simulink model "bp_attitude_control"  (R2024b)
settings: Solver=FixedStepAuto  StartTime=0.0  StopTime=1000  FixedStep=1  RelTol=1e-3
values from neighbouring files (symbols this model uses):
  H0 = [30; 30; 30]    [initialcondition.m]
  I = [1759 0 0; 0 2758 0; 0 0 2171]    [initialcondition.m]
  qZYX = eul2quat(Euler0)    [initialcondition.m]
  w0 = [0; 0; 0]    [initialcondition.m]
settings Model: Creator=ThinkBook  LastModifiedBy=Lzy18
settings DebuggingCC: UnconnectedInputMsg=warning  UnconnectedOutputMsg=warning  UnconnectedLineMsg=warning
settings ModelReferenceCC: EnableRefExpFcnMdlSchedulingChecks=on
settings RTWCC: GPUComputeCapability=3.5  DLArmComputeVersion=19.05

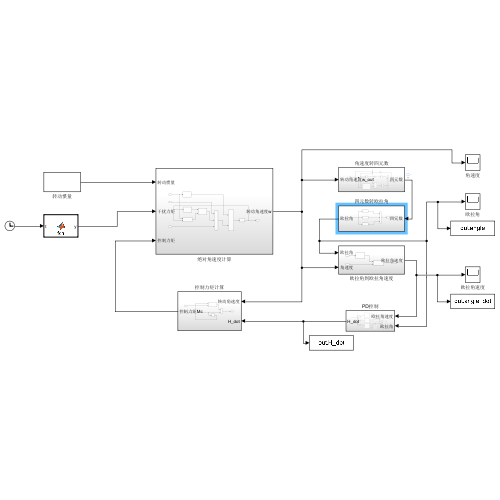
[thumbnail: Simulink's stored preview of the top-level diagram]
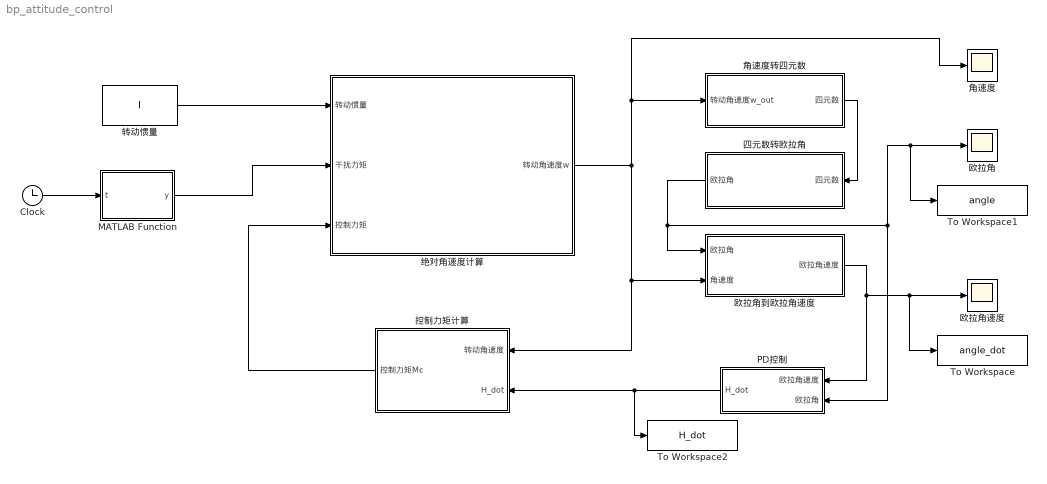
== system bp_attitude_control ==
  Clock : Clock
  MATLAB Function : MATLAB Function  TreatAsAtomicUnit=on
  PD控制 : Subsystem
  To Workspace : ToWorkspace  VariableName=angle_dot  SampleTime=-1
  To Workspace1 : ToWorkspace  VariableName=angle  SampleTime=-1
  To Workspace2 : ToWorkspace  VariableName=H_dot  SampleTime=-1
  四元数转欧拉角 : Subsystem
  控制力矩计算 : Subsystem
  欧拉角 : Scope
  欧拉角到欧拉角速度 : Subsystem
  欧拉角速度 : Scope
  绝对角速度计算 : Subsystem
  角速度 : Scope
  角速度转四元数 : Subsystem
  转动惯量 : Constant  Value=I
  wires:
  转动惯量/1 -> 绝对角速度计算/1(转动惯量)
  控制力矩计算/1(控制力矩Mc) -> 绝对角速度计算/3(控制力矩)
  绝对角速度计算/1(转动角速度w) -> 角速度/1, 角速度转四元数/1(转动角速度w_out), 控制力矩计算/1(转动角速度), 欧拉角到欧拉角速度/2(角速度)
  角速度转四元数/1(四元数) -> 四元数转欧拉角/1(四元数)
  四元数转欧拉角/1(欧拉角) -> 欧拉角到欧拉角速度/1(欧拉角), PD控制/2(欧拉角), To Workspace1/1, 欧拉角/1
  MATLAB Function/1(y) -> 绝对角速度计算/2(干扰力矩)
  Clock/1 -> MATLAB Function/1(t)
  欧拉角到欧拉角速度/1(欧拉角速度) -> PD控制/1(欧拉角速度), To Workspace/1, 欧拉角速度/1
  PD控制/1(H_dot) -> To Workspace2/1, 控制力矩计算/2(H_dot)

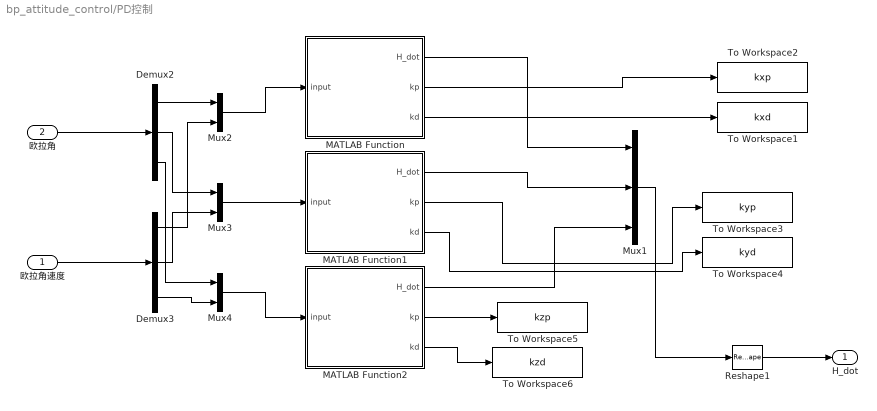
== system bp_attitude_control/PD控制 ==
  欧拉角速度 : Inport
  欧拉角 : Inport  Port=2
  Demux2 : Demux  Outputs=3
  Demux3 : Demux  Outputs=3
  MATLAB Function : MATLAB Function  TreatAsAtomicUnit=on
  MATLAB Function1 : MATLAB Function  TreatAsAtomicUnit=on
  MATLAB Function2 : MATLAB Function  TreatAsAtomicUnit=on
  Mux1 : Mux  Inputs=3
  Mux2 : Mux  Inputs=2
  Mux3 : Mux  Inputs=2
  Mux4 : Mux  Inputs=2
  Reshape1 : Reshape  OutputDimensionality=Customize  OutputDimensions=[3,1]
  To Workspace1 : ToWorkspace  VariableName=kxd  SampleTime=-1
  To Workspace2 : ToWorkspace  VariableName=kxp  SampleTime=-1
  To Workspace3 : ToWorkspace  VariableName=kyp  SampleTime=-1
  To Workspace4 : ToWorkspace  VariableName=kyd  SampleTime=-1
  To Workspace5 : ToWorkspace  VariableName=kzp  SampleTime=-1
  To Workspace6 : ToWorkspace  VariableName=kzd  SampleTime=-1
  H_dot : Outport
  wires:
  欧拉角速度/1 -> Demux3/1
  欧拉角/1 -> Demux2/1
  Mux1/1 -> Reshape1/1
  Reshape1/1 -> H_dot/1
  MATLAB Function/1(H_dot) -> Mux1/1
  MATLAB Function1/1(H_dot) -> Mux1/2
  MATLAB Function2/1(H_dot) -> Mux1/3
  MATLAB Function/2(kp) -> To Workspace2/1
  MATLAB Function/3(kd) -> To Workspace1/1
  MATLAB Function1/2(kp) -> To Workspace3/1
  MATLAB Function1/3(kd) -> To Workspace4/1
  MATLAB Function2/2(kp) -> To Workspace5/1
  MATLAB Function2/3(kd) -> To Workspace6/1
  Demux2/1 -> Mux2/1
  Demux3/1 -> Mux2/2
  Mux2/1 -> MATLAB Function/1(input)
  Demux2/2 -> Mux3/1
  Demux3/2 -> Mux3/2
  Mux3/1 -> MATLAB Function1/1(input)
  Demux2/3 -> Mux4/1
  Demux3/3 -> Mux4/2
  Mux4/1 -> MATLAB Function2/1(input)

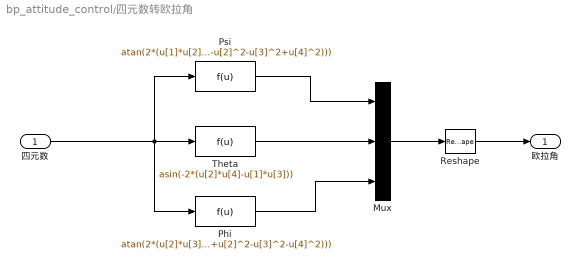
== system bp_attitude_control/四元数转欧拉角 ==
  四元数 : Inport
  Mux : Mux  Inputs=3
  Phi : Fcn  Expr=atan(2*(u[2]*u[3]+u[1]*u[4]/(u[1]^2+u[2]^2-u[3]^2-u[4]^2)))
  Psi : Fcn  Expr=atan(2*(u[1]*u[2]+u[3]*u[4]/(u[1]^2-u[2]^2-u[3]^2+u[4]^2)))
  Reshape : Reshape  OutputDimensionality=Customize  OutputDimensions=[3,1]
  Theta : Fcn  Expr=asin(-2*(u[2]*u[4]-u[1]*u[3]))
  欧拉角 : Outport
  wires:
  Psi/1 -> Mux/1
  四元数/1 -> Phi/1, Psi/1, Theta/1
  Theta/1 -> Mux/2
  Phi/1 -> Mux/3
  Mux/1 -> Reshape/1
  Reshape/1 -> 欧拉角/1

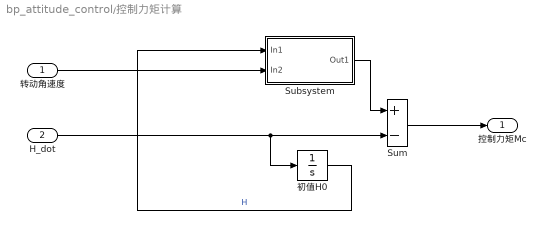
== system bp_attitude_control/控制力矩计算 ==
  转动角速度 : Inport
  H_dot : Inport  Port=2
  Subsystem : Subsystem
      mask Display:
      | disp('Cross \nProduct')
      | port_label('input',1,'X')
      | port_label('input',2,'Y')
      | port_label('output',1,'X*Y')
  Sum : Sum  Inputs=+-
  初值H0 : Integrator  InitialCondition=H0
  控制力矩Mc : Outport
  wires:
  Sum/1 -> 控制力矩Mc/1
  转动角速度/1 -> Subsystem/2(In2)
  H_dot/1 -> Sum/2, 初值H0/1
  Subsystem/1(Out1) -> Sum/1
  初值H0/1 -> Subsystem/1(In1)  "H"

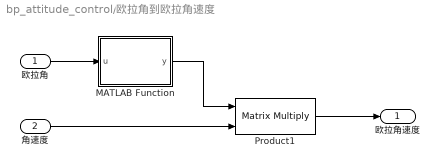
== system bp_attitude_control/欧拉角到欧拉角速度 ==
  欧拉角 : Inport
  角速度 : Inport  Port=2
  MATLAB Function : MATLAB Function  TreatAsAtomicUnit=on
  Product1 : Product  Multiplication=Matrix(*)
  欧拉角速度 : Outport
  wires:
  Product1/1 -> 欧拉角速度/1
  欧拉角/1 -> MATLAB Function/1(u)
  MATLAB Function/1(y) -> Product1/1
  角速度/1 -> Product1/2

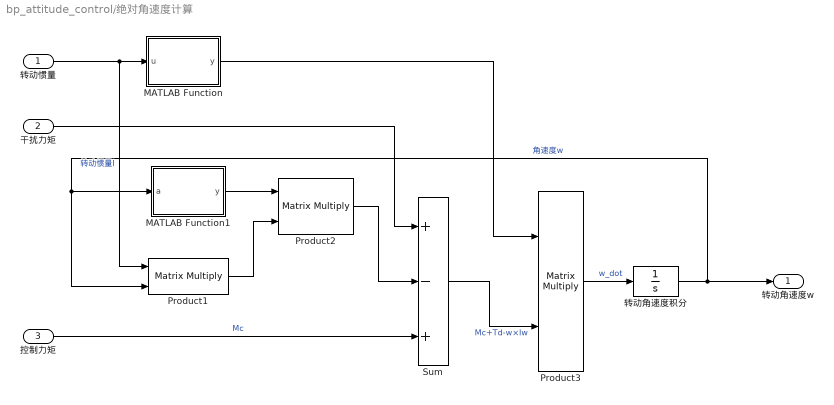
== system bp_attitude_control/绝对角速度计算 ==
  转动惯量 : Inport
  干扰力矩 : Inport  Port=2
  控制力矩 : Inport  Port=3
  MATLAB Function : MATLAB Function  TreatAsAtomicUnit=on
  MATLAB Function1 : MATLAB Function  TreatAsAtomicUnit=on
  Product1 : Product  Multiplication=Matrix(*)
  Product2 : Product  Multiplication=Matrix(*)
  Product3 : Product  Multiplication=Matrix(*)
  Sum : Sum  Inputs=+-+
  转动角速度积分 : Integrator  InitialCondition=w0
  转动角速度w : Outport
  wires:
  Sum/1 -> Product3/2  "Mc+Td-w×Iw"
  Product3/1 -> 转动角速度积分/1  "w_dot"
  转动角速度积分/1 -> Product1/2, MATLAB Function1/1(a), 转动角速度w/1  "角速度w"
  转动惯量/1 -> MATLAB Function/1(u), Product1/1  "转动惯量I"
  控制力矩/1 -> Sum/3  "Mc"
  MATLAB Function/1(y) -> Product3/1
  MATLAB Function1/1(y) -> Product2/1
  Product1/1 -> Product2/2
  Product2/1 -> Sum/2
  干扰力矩/1 -> Sum/1

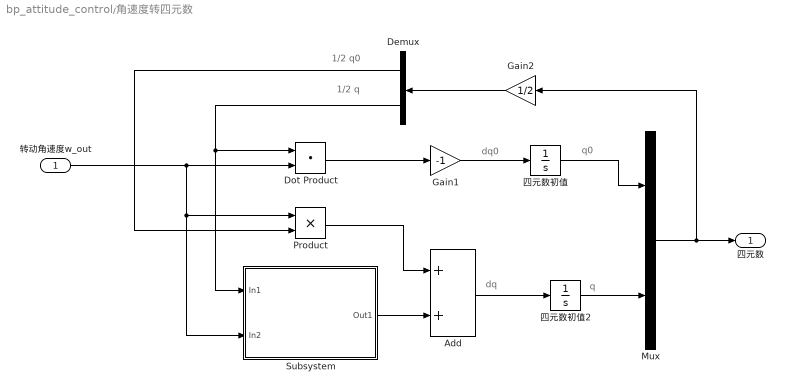
== system bp_attitude_control/角速度转四元数 ==
  note: q
  note: dq
  note: dq0
  note: q0
  note: 1/2 q0
  note: 1/2 q
  转动角速度w_out : Inport
  Add : Sum
  Demux : Demux  Outputs=2
  Dot Product : DotProduct  OutDataTypeStr=Inherit: Inherit via internal rule
  Gain1 : Gain  Gain=-1
  Gain2 : Gain  Gain=1/2
  Mux : Mux  Inputs=[1 3]
  Product : Product
  Subsystem : Subsystem
      mask Display:
      | disp('Cross \nProduct')
      | port_label('input',1,'X')
      | port_label('input',2,'Y')
      | port_label('output',1,'X*Y')
  四元数初值 : Integrator  InitialCondition=qZYX(1)
  四元数初值2 : Integrator  InitialCondition=qZYX(2:4)'
  四元数 : Outport
  wires:
  Demux/2 -> Dot Product/1, Subsystem/1(In1)
  Gain1/1 -> 四元数初值/1
  Subsystem/1(Out1) -> Add/2
  四元数初值/1 -> Mux/1
  Demux/1 -> Product/2
  Gain2/1 -> Demux/1
  Mux/1 -> Gain2/1, 四元数/1
  转动角速度w_out/1 -> Product/1, Subsystem/2(In2), Dot Product/2
  Add/1 -> 四元数初值2/1
  Dot Product/1 -> Gain1/1
  四元数初值2/1 -> Mux/2
  Product/1 -> Add/1

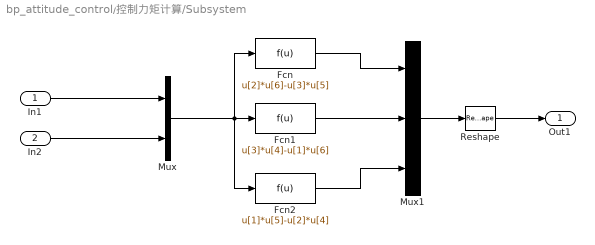
== system bp_attitude_control/控制力矩计算/Subsystem ==
  In1 : Inport
  In2 : Inport  Port=2
  Fcn : Fcn  Expr=u[2]*u[6]-u[3]*u[5]
  Fcn1 : Fcn  Expr=u[3]*u[4]-u[1]*u[6]
  Fcn2 : Fcn  Expr=u[1]*u[5]-u[2]*u[4]
  Mux : Mux  Inputs=2
  Mux1 : Mux  Inputs=3
  Reshape : Reshape  OutputDimensionality=Customize  OutputDimensions=[3,1]
  Out1 : Outport
  wires:
  In2/1 -> Mux/2
  In1/1 -> Mux/1
  Fcn/1 -> Mux1/1
  Fcn1/1 -> Mux1/2
  Fcn2/1 -> Mux1/3
  Mux/1 -> Fcn2/1, Fcn/1, Fcn1/1
  Reshape/1 -> Out1/1
  Mux1/1 -> Reshape/1

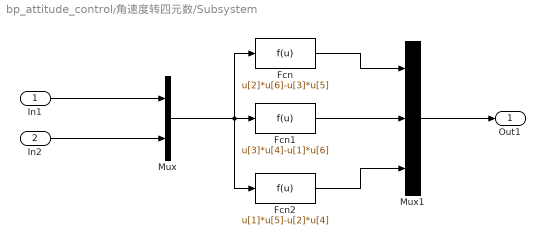
== system bp_attitude_control/角速度转四元数/Subsystem ==
  In1 : Inport
  In2 : Inport  Port=2
  Fcn : Fcn  Expr=u[2]*u[6]-u[3]*u[5]
  Fcn1 : Fcn  Expr=u[3]*u[4]-u[1]*u[6]
  Fcn2 : Fcn  Expr=u[1]*u[5]-u[2]*u[4]
  Mux : Mux  Inputs=2
  Mux1 : Mux  Inputs=3
  Out1 : Outport
  wires:
  In2/1 -> Mux/2
  In1/1 -> Mux/1
  Fcn/1 -> Mux1/1
  Fcn1/1 -> Mux1/2
  Fcn2/1 -> Mux1/3
  Mux/1 -> Fcn2/1, Fcn/1, Fcn1/1
  Mux1/1 -> Out1/1

== matlab function bp_attitude_control/欧拉角到欧拉角速度/MATLAB Function ==
  data: u input; y output
function y = fcn(u)
Psi = u(1);
Theta = u(2);

y = [1 sin(Psi)*tan(Theta) cos(Psi)*tan(Theta);
    0 cos(Psi) -sin(Psi);
    0 sin(Psi)/cos(Theta) cos(Psi)/cos(Theta)];

end

== matlab function bp_attitude_control/绝对角速度计算/MATLAB Function ==
  data: u input; y output
function y = fcn(u)

y = inv(u);

end

== matlab function bp_attitude_control/绝对角速度计算/MATLAB Function1 ==
  data: a input; y output
function y = fcn(a)
% Convert input vectors to 3x3 matrices
A=[0 -a(3) a(2);a(3) 0 -a(1);-a(2) a(1) 0];
% Calculate cross product of matrices
y=A;
end

== matlab function bp_attitude_control/MATLAB Function ==
  data: t input; y output
function y = fcn(t)
w = 3;
y = [1*sin(w*t);
     2*cos(w*t+pi/3); 
     3*cos(w*t)];
end

== matlab function bp_attitude_control/PD控制/MATLAB Function ==
  settings: updateMethod=DISCRETE
  data: input input; H_dot output; kp output; kd output
function [H_dot, kp, kd] = BP_PD(input)
    persistent wi wo wi_1 wo_1 wi_2 wo_2 du_1 y error Oh M xite alfa IN H Out;

    if isempty(wi)
        % 初始化权值参数
        IN = 3;  % 输入层节点数
        H = 4 ;   % 隐层节点数
        Out = 2;  % 输出层节点数

        xite = 0.75;  % 学习率
        alfa = 0.05;  % 动量因子
        
        wi = 0.50 * rand(H, IN);  % 输入到隐层的权重
        wo = 0.50 * rand(Out, H);  % 隐层到输出层的权重
        
        % 权重历史
        wo_1 = wo;  
        wo_2 = wo; 
        wi_1 = wi;  
        wi_2 = wi;

        % PID控制器参数
        M = [10.2435, 394.7569];  % PID增益系数
        
        % 初始化变量
        du_1 = 0;       % 上一次的控制量
        y = zeros(1, 3); % 系统输出
        error = zeros(1, 2); % 误差历史
        Oh = zeros(H, 1);  % 隐层输出
    end

    X = zeros(1, 2);
    dK = zeros(1,Out);
    delta3 = zeros(1, Out);
    delta2 = zeros(1, H);
    
    angle = input(1);
    angle_dot = input(2);

    rin = angle;            % 输入值
    yout = 0;              % 目标值
    error(1) = rin - yout; % 计算误差

    % 误差变化率和历史误差
    X(1) = angle; 
    X(2) = angle_dot; 

    xii = [X(1), X(2), 0.01];  % 输入向量，加上偏置项
    norm_xii = norm(xii);
    
    if norm_xii ~= 0
        xi = xii / norm_xii;  % 归一化输入
    else
        xi = xii;  % 避免除以零
    end
    
    epid = [X(1); X(2)];    % PID控制器输入

    % 前向传播----------------------------------------
    net2 = xi * (wi');  % 计算隐层输入
    for j = 1:H
        Oh(j) = tanh(net2(j));  % 隐层输出
    end

    net3 = wo * Oh;  % 计算输出层输入
    K = 1 ./ (1 + exp(-net3));  % 输出

    kp = M(1) * K(1); 
    kd = M(2) * K(2); 

    du = kp * X(1) + kd * X(2);   % 控制量变化
    du = max(min(du, 10), -10);  % 将控制量限制在[-10, 10]

    % 反向传播更新权值------------------------------------------------
    dyu = sign((yout - y(1)) / (du - du_1 + 0.0001));  % 计算输出变化方向
    for j = 1:Out
        dK(j) = K(j) * (1 - K(j));  % sigmoid的梯度
    end

    for l = 1:Out
        delta3(l) = error(1) * dyu * epid(l) * dK(l);  % 输出层误差
    end

    d_wo = zeros(Out, H);  % 初始化权重变化
    for l = 1:Out
        for i = 1:H
            d_wo(l, i) = xite * delta3(l) * Oh(i);  % 计算输出权重变化
        end
    end
    wo = wo_1 + d_wo + alfa * (wo_1 - wo_2);  % 更新输出层权重

    dO = zeros(H, 1);
    for i = 1:H
        dO(i) = 1 - Oh(i)^2;  % tanh的导数
    end
    segma = delta3 * wo;  % 计算隐层误差
    for i = 1:H
        delta2(i) = dO(i) * segma(i);  % 隐层误差
    end
    d_wi = xite * delta2' * xi;  % 计算输入权重变化
    wi = wi_1 + d_wi + alfa * (wi_1 - wi_2);  % 更新输入层权重

    wo_2 = wo_1; 
    wo_1 = wo;
    wi_2 = wi_1; 
    wi_1 = wi;

    du_1 = du;   
    H_dot = kp * angle + kd * angle_dot;  % 返回控制输出
end

== matlab function bp_attitude_control/PD控制/MATLAB Function1 ==
  settings: updateMethod=DISCRETE
  data: input input; H_dot output; kp output; kd output
function [H_dot, kp, kd] = BP_PD(input)
    persistent wi wo wi_1 wo_1 wi_2 wo_2 du_1 y error Oh M xite alfa IN H Out;

    if isempty(wi)
        % 初始化权值参数
        IN = 3;  % 输入层节点数
        H = 4 ;   % 隐层节点数
        Out = 2;  % 输出层节点数

        xite = 0.75;  % 学习率
        alfa = 0.05;  % 动量因子
        
        wi = 0.50 * rand(H, IN);  % 输入到隐层的权重
        wo = 0.50 * rand(Out, H);  % 隐层到输出层的权重
        
        % 权重历史
        wo_1 = wo;  
        wo_2 = wo; 
        wi_1 = wi;  
        wi_2 = wi;

        % PID控制器参数
        M = [2.3318, 165.8386];  % PID增益系数
        
        % 初始化变量
        du_1 = 0;       % 上一次的控制量
        y = zeros(1, 3); % 系统输出
        error = zeros(1, 2); % 误差历史
        Oh = zeros(H, 1);  % 隐层输出
    end

    X = zeros(1, 2);
    dK = zeros(1,Out);
    delta3 = zeros(1, Out);
    delta2 = zeros(1, H);
    
    angle = input(1);
    angle_dot = input(2);

    rin = angle;            % 输入值
    yout = 0;              % 目标值
    error(1) = rin - yout; % 计算误差

    % 误差变化率和历史误差
    X(1) = angle; 
    X(2) = angle_dot; 

    xii = [X(1), X(2), 0.01];  % 输入向量，加上偏置项
    norm_xii = norm(xii);
    
    if norm_xii ~= 0
        xi = xii / norm_xii;  % 归一化输入
    else
        xi = xii;  % 避免除以零
    end
    
    epid = [X(1); X(2)];    % PID控制器输入

    % 前向传播----------------------------------------
    net2 = xi * (wi');  % 计算隐层输入
    for j = 1:H
        Oh(j) = tanh(net2(j));  % 隐层输出
    end

    net3 = wo * Oh;  % 计算输出层输入
    K = 1 ./ (1 + exp(-net3));  % 输出

    kp = M(1) * K(1); 
    kd = M(2) * K(2); 

    du = kp * X(1) + kd * X(2);   % 控制量变化
    du = max(min(du, 10), -10);  % 将控制量限制在[-10, 10]

    % 反向传播更新权值------------------------------------------------
    dyu = sign((yout - y(1)) / (du - du_1 + 0.0001));  % 计算输出变化方向
    for j = 1:Out
        dK(j) = K(j) * (1 - K(j));  % sigmoid的梯度
    end

    for l = 1:Out
        delta3(l) = error(1) * dyu * epid(l) * dK(l);  % 输出层误差
    end

    d_wo = zeros(Out, H);  % 初始化权重变化
    for l = 1:Out
        for i = 1:H
            d_wo(l, i) = xite * delta3(l) * Oh(i);  % 计算输出权重变化
        end
    end
    wo = wo_1 + d_wo + alfa * (wo_1 - wo_2);  % 更新输出层权重

    dO = zeros(H, 1);
    for i = 1:H
        dO(i) = 1 - Oh(i)^2;  % tanh的导数
    end
    segma = delta3 * wo;  % 计算隐层误差
    for i = 1:H
        delta2(i) = dO(i) * segma(i);  % 隐层误差
    end
    d_wi = xite * delta2' * xi;  % 计算输入权重变化
    wi = wi_1 + d_wi + alfa * (wi_1 - wi_2);  % 更新输入层权重

    wo_2 = wo_1; 
    wo_1 = wo;
    wi_2 = wi_1; 
    wi_1 = wi;

    du_1 = du;   
    H_dot = kp * angle + kd * angle_dot;  % 返回控制输出
end

== matlab function bp_attitude_control/PD控制/MATLAB Function2 ==
  settings: updateMethod=DISCRETE
  data: input input; H_dot output; kp output; kd output
function [H_dot, kp, kd] = BP_PD(input)
    persistent wi wo wi_1 wo_1 wi_2 wo_2 du_1 y error Oh M xite alfa IN H Out;

    if isempty(wi)
        % 初始化权值参数
        IN = 3;  % 输入层节点数
        H = 4 ;   % 隐层节点数
        Out = 2;  % 输出层节点数

        xite = 0.75;  % 学习率
        alfa = 0.05;  % 动量因子
        
        wi = 0.50 * rand(H, IN);  % 输入到隐层的权重
        wo = 0.50 * rand(Out, H);  % 隐层到输出层的权重
        
        % 权重历史
        wo_1 = wo;  
        wo_2 = wo; 
        wi_1 = wi;  
        wi_2 = wi;

        % PID控制器参数
        M = [11.1317, 636.8378];  % PID增益系数
        
        % 初始化变量
        du_1 = 0;       % 上一次的控制量
        y = zeros(1, 3); % 系统输出
        error = zeros(1, 2); % 误差历史
        Oh = zeros(H, 1);  % 隐层输出
    end

    X = zeros(1, 2);
    dK = zeros(1,Out);
    delta3 = zeros(1, Out);
    delta2 = zeros(1, H);
    
    angle = input(1);
    angle_dot = input(2);

    rin = angle;            % 输入值
    yout = 0;              % 目标值
    error(1) = rin - yout; % 计算误差

    % 误差变化率和历史误差
    X(1) = angle; 
    X(2) = angle_dot; 

    xii = [X(1), X(2), 0.01];  % 输入向量，加上偏置项
    norm_xii = norm(xii);
    
    if norm_xii ~= 0
        xi = xii / norm_xii;  % 归一化输入
    else
        xi = xii;  % 避免除以零
    end
    
    epid = [X(1); X(2)];    % PID控制器输入

    % 前向传播----------------------------------------
    net2 = xi * (wi');  % 计算隐层输入
    for j = 1:H
        Oh(j) = tanh(net2(j));  % 隐层输出
    end

    net3 = wo * Oh;  % 计算输出层输入
    K = 1 ./ (1 + exp(-net3));  % 输出

    kp = M(1) * K(1); 
    kd = M(2) * K(2); 

    du = kp * X(1) + kd * X(2);   % 控制量变化
    du = max(min(du, 10), -10);  % 将控制量限制在[-10, 10]

    % 反向传播更新权值------------------------------------------------
    dyu = sign((yout - y(1)) / (du - du_1 + 0.0001));  % 计算输出变化方向
    for j = 1:Out
        dK(j) = K(j) * (1 - K(j));  % sigmoid的梯度
    end

    for l = 1:Out
        delta3(l) = error(1) * dyu * epid(l) * dK(l);  % 输出层误差
    end

    d_wo = zeros(Out, H);  % 初始化权重变化
    for l = 1:Out
        for i = 1:H
            d_wo(l, i) = xite * delta3(l) * Oh(i);  % 计算输出权重变化
        end
    end
    wo = wo_1 + d_wo + alfa * (wo_1 - wo_2);  % 更新输出层权重

    dO = zeros(H, 1);
    for i = 1:H
        dO(i) = 1 - Oh(i)^2;  % tanh的导数
    end
    segma = delta3 * wo;  % 计算隐层误差
    for i = 1:H
        delta2(i) = dO(i) * segma(i);  % 隐层误差
    end
    d_wi = xite * delta2' * xi;  % 计算输入权重变化
    wi = wi_1 + d_wi + alfa * (wi_1 - wi_2);  % 更新输入层权重

    wo_2 = wo_1; 
    wo_1 = wo;
    wi_2 = wi_1; 
    wi_1 = wi;

    du_1 = du;   
    H_dot = kp * angle + kd * angle_dot;  % 返回控制输出
end
